simulink model "gradiente_normalizado"  (Simulink 10.3)
settings: Solver=ode45  StartTime=10  StopTime=20  RelTol=1e-3  AbsTol=1e-6
values from neighbouring files (symbols this model uses):
  As = 2    [sim_grad_norm_n2.m]    (also in simu01.m)
  DC = 1    [sim_grad_norm_n2.m]    (also in simu01.m)
  gamma = gamma1    [sim_grad_norm_n2.m]    (also in simu01.m)
  kappa = 0    [sim_grad_norm_n2.m]    (also in simu01.m)
  lambda0 = 1    [sim_grad_norm_n2.m]    (also in simu01.m)
  lambda1 = 2    [sim_grad_norm_n2.m]    (also in simu01.m)
  st = 0.01    [sim_grad_norm_n2.m]    (also in simu01.m)
  theta0 = [0;0;0;0]    [sim_grad_norm_n2.m]    (also in simu01.m)
  thetas = [b0; b1; a0; a1]    [simu01.m]
  ws = 0.1*pi    (= 0.314159265359)    [sim_grad_norm_n2.m]    (also in simu01.m)
libraries: cstblocks x1
settings Model: Creator=Ramon  LastModifiedBy=Lucas  MultithreadedSim=on
settings SolverCC: AutoScaleAbsTol=off
settings DataIOCC: SaveOutput=off  SaveTime=off
settings OptimizationCC: BlockReduction=off  BooleanDataType=off  InitFltsAndDblsToZero=on
settings DebuggingCC: SaveWithParameterizedLinksMsg=none  SignalResolutionControl=TryResolveAllWithWarning  MultiTaskDSMMsg=warning  MultiTaskCondExecSysMsg=none
settings HardwareCC: TargetUnknown=on
settings RTWCC: TemplateMakefile=grt_vc.tmf

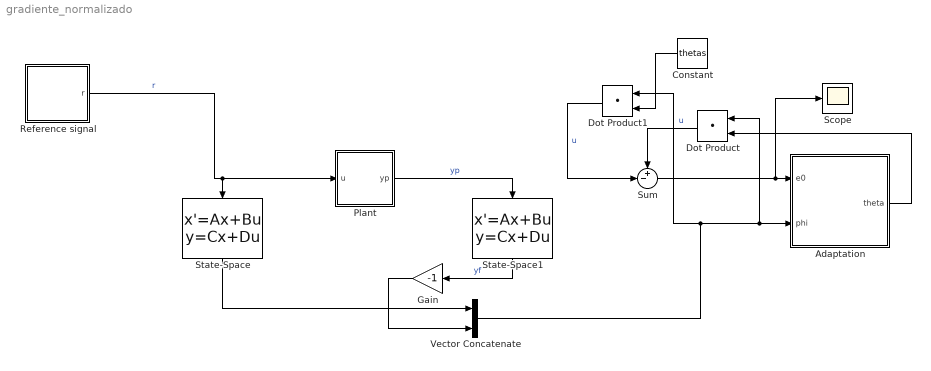
== system gradiente_normalizado ==
  Adaptation : Subsystem
  Constant : Constant  Value=thetas
  Dot Product : DotProduct  InputSameDT=on  OutDataTypeStr=Inherit: Inherit via internal rule
  Dot Product1 : DotProduct  InputSameDT=on  OutDataTypeStr=Inherit: Inherit via internal rule
  Gain : Gain  Gain=-1
  Plant : Subsystem
  Reference signal : Subsystem
  Scope : Scope
  State-Space : StateSpace  A=[0 1; -lambda0 -lambda1]  B=[0; 1]  C=[1 0;0 1]  D=[0; 0]  InitialCondition=0
  State-Space1 : StateSpace  A=[0 1; -lambda0 -lambda1]  B=[0; 1]  C=[1 0;0 1]  D=[0; 0]  InitialCondition=0
  Sum : Sum  Inputs=+-|
  Vector Concatenate : Concatenate
  wires:
  Adaptation/1(theta) -> Dot Product/2
  Vector Concatenate/1 -> Adaptation/2(phi), Dot Product/1, Dot Product1/1
  Reference signal/1(r) -> State-Space/1, Plant/1(u)  "r"
  Plant/1(yp) -> State-Space1/1  "yp"
  State-Space1/1 -> Gain/1  "yf"
  State-Space/1 -> Vector Concatenate/1
  Gain/1 -> Vector Concatenate/2
  Sum/1 -> Scope/1, Adaptation/1(e0)
  Dot Product/1 -> Sum/1  "u"
  Constant/1 -> Dot Product1/2
  Dot Product1/1 -> Sum/2  "u"

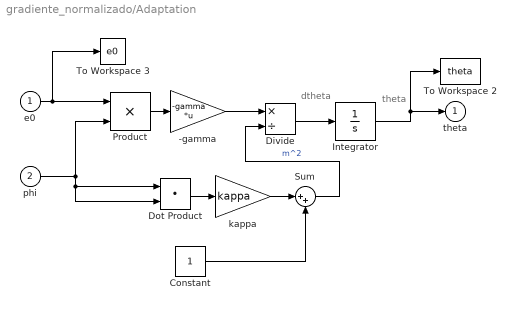
== system gradiente_normalizado/Adaptation ==
  note: theta
  note: dtheta
  e0 : Inport  PortDimensions=1
  phi : Inport  Port=2
  -gamma : Gain  Gain=-gamma  Multiplication=Matrix(K*u) (u vector)  SaturateOnIntegerOverflow=on  OutDataTypeStr=Inherit: Same as input  ParamDataTypeStr=Inherit: Same as input
  Constant : Constant
  Divide : Product  Inputs=*/
  Dot Product : DotProduct  InputSameDT=on  OutDataTypeStr=Inherit: Inherit via internal rule
  Integrator : Integrator  InitialCondition=theta0
  Product : Product  InputSameDT=on  RndMeth=Zero  SaturateOnIntegerOverflow=on  OutDataTypeStr=Inherit: Same as first input
  Sum : Sum  Inputs=|++
  To Workspace 2 : ToWorkspace  VariableName=theta  SampleTime=st
  To Workspace 3 : ToWorkspace  VariableName=e0  SampleTime=st
  kappa : Gain  Gain=kappa  SaturateOnIntegerOverflow=on  OutDataTypeStr=Inherit: Same as input  ParamDataTypeStr=Inherit: Same as input
  theta : Outport  InitialOutput=0  VectorParamsAs1DForOutWhenUnconnected=off
  wires:
  Integrator/1 -> To Workspace 2/1, theta/1
  Divide/1 -> Integrator/1
  phi/1 -> Product/2, Dot Product/2, Dot Product/1
  e0/1 -> Product/1, To Workspace 3/1
  -gamma/1 -> Divide/1
  Product/1 -> -gamma/1
  Dot Product/1 -> kappa/1
  Constant/1 -> Sum/2
  kappa/1 -> Sum/1
  Sum/1 -> Divide/2  "m^2"

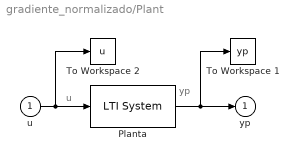
== system gradiente_normalizado/Plant ==
  note: yp
  note: u
  u : Inport
  Planta : cstblocks/LTI System  sys=P  IC=x0
  To Workspace 1 : ToWorkspace  VariableName=yp  SampleTime=st
  To Workspace 2 : ToWorkspace  VariableName=u  SampleTime=st
  yp : Outport  InitialOutput=0  VectorParamsAs1DForOutWhenUnconnected=off
  wires:
  u/1 -> To Workspace 2/1, Planta/1
  Planta/1 -> yp/1, To Workspace 1/1

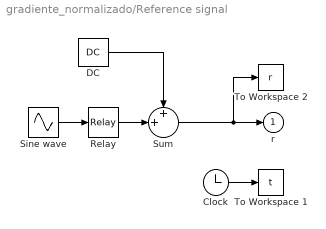
== system gradiente_normalizado/Reference signal ==
  Clock : Clock
  DC : Constant  Value=DC
  Relay : Relay  OnOutputValue=As  OffOutputValue=-As
  Sine wave : Sin  Frequency=ws  SampleTime=0
  Sum : Sum  Inputs=++|  InputSameDT=on  SaturateOnIntegerOverflow=on  OutDataTypeStr=Inherit: Same as first input
  To Workspace 1 : ToWorkspace  VariableName=t  SampleTime=st
  To Workspace 2 : ToWorkspace  VariableName=r  SampleTime=st
  r : Outport  InitialOutput=0  VectorParamsAs1DForOutWhenUnconnected=off
  wires:
  DC/1 -> Sum/1
  Sum/1 -> r/1, To Workspace 2/1
  Clock/1 -> To Workspace 1/1
  Sine wave/1 -> Relay/1
  Relay/1 -> Sum/2
